simulink model "Vehicle_Model_999_Modular_roll_gradient"  (R2025b)
settings: Solver=ode23tb  StartTime=0.0  StopTime=72  MaxStep=0.001  RelTol=1e-3
values from neighbouring files (symbols this model uses):
  aero_par = struct()    [Load_aero_parameters.m]
  Ki_array = zeros(size(Vx_array))    [Torque_vectoring_workspace_lookuptable_v2.m]
  Kp_array = zeros(size(Vx_array))    [Torque_vectoring_workspace_lookuptable_v2.m]
  ku = (lr*m*9.81/(cf*(lf+lr))) - (lf*m*9.81/(cr*(lf+lr)))    (= -0.00172747958109)    [Torque_vectoring_workspace_lookuptable_v2.m]
  m = Par.m    [Lapsim_Endurance_inverse_v3.m]    (also in New_LapSim_final_ts_v1.m = Par.Mass; Rajdeep_sus_scriptv2.m = 270; Torque_vectoring_workspace_lookuptable_v2.m = 270)
  Par = struct()    [Load_vehicle_parameters.m]
  path_Theta = theta-theta_0    [New_LapSim_final_ts_v1.m]
  sus_par = struct()    [Load_sus_parameters.m]
  TireData = Tir    [prep_tire_data.m]
  Vx_array = 1:1:21    [Torque_vectoring_workspace_lookuptable_v2.m]
undefined symbols (not defined in the file or in its folder): additional_steering, Battery, Brake_Val, ctrl_Brake, ctrl_s, ctrl_Steer, ctrl_Throttle, ctrl_Velocity, HP, init_r, init_vx, init_vy, Motor, path_X, path_Y, skidpad_time, skidpad_vel, steer_input, Steer_Val, TC_target_slip, Throttle_Val, V_ref
libraries: simulink x16, autolibshared x3, simulink_extras x2, BatteryEstimators x1
(part 4 of 4)

== matlab function Vehicle_Model_999_Modular_roll_gradient/Vehicle dynamics/Fx, Fy calculations with grip limit/Grip_limit/MATLAB Function1 ==
  data: Fx input; Fx_new output; Fy input; Dx input; Dy input; s input; Fy_new output
function [Fx_new, Fy_new] = fcn(Fx, Fy, Dx, Dy, s)
    % Initialize outputs
    Fx_new = Fx;
    Fy_new = Fy;
    
    if s > 1
        % 1. Add a tiny protection value (1e-6) to prevent divide-by-zero
        Dx_safe = max(abs(Dx), 1e-3);
        Dy_safe = max(abs(Dy), 1e-3);
        
        % 2. Calculate the grip saturation (eta) for all tires
        eta = sqrt((Fx ./ Dx_safe).^2 + (Fy ./ Dy_safe).^2);
        
        % 3. Find the indices of the tires that are exceeding 100% grip
        over_limit_idx = eta > 1;
        
        % 4. Proportionally scale down ONLY the tires that are slipping
        % This scales the vector perfectly to the edge of the ellipse 
        % without changing the force direction.
        Fx_new(over_limit_idx) = Fx(over_limit_idx) ./ eta(over_limit_idx);
        Fy_new(over_limit_idx) = Fy(over_limit_idx) ./ eta(over_limit_idx);
    end
end

== matlab function Vehicle_Model_999_Modular_roll_gradient/E-powertrain/Motor/rpm selection for third wheel ==
  data: u input; y output
function y = fcn(u)

y = u(3);

== matlab function Vehicle_Model_999_Modular_roll_gradient/Inputs/steer_input_simulink/MATLAB Function ==
  settings: updateMethod=DISCRETE
  data: X input; delta output; Y input; PSI input; vx input; vy input; path_Y input; path_X input; path_Theta input
function delta = get_steering_command(X, Y, PSI, vx,vy,path_Y, path_X, path_Theta)
    % GET_STEERING_COMMAND Simulink-safe Stanley implementation
   
    %% Parameters
    L_f = 0.78132;          % Pre-multiplied 1.532 * 0.51 for efficiency
    v_eps = 1.0;            % Softening constant to prevent singularity
    v_switch = 5.0;         % Velocity threshold for slip compensation (m/s)
    max_steer = deg2rad(25);% Physical steering limit
    k_stanley = 0;
    %% 1. Sensing (Shift to Front Axle)
    xf = X + L_f * cos(PSI); 
    yf = Y + L_f * sin(PSI);
    
    %% 2. Global Nearest Point Search (Fixed-Size for Simulink)
    % Calculate squared distances to ALL points to maintain fixed array sizes
    dx = path_X - xf;
    dy = path_Y - yf;
    distances = dx.^2 + dy.^2; 
    
    [~, idx_closest] = min(distances);
    Npath = length(path_X);
    
    % %% 3. Path Heading Calculation
    % if Npath <= 1
    %     % Failsafe: If the path is only 1 point, we cannot calculate a slope.
    %     % Default to 0, or you could output an error flag.
    %     path_Theta = 0; 
    % elseif idx_closest < Npath
    %     % Forward difference (standard operation)
    %     path_Theta = atan2(path_X(idx_closest+1) - path_X(idx_closest),path_Y(idx_closest+1) - path_Y(idx_closest));
    % else
    %     % Backward difference (only triggers when exactly on the final point of the track)
    %     path_Theta = atan2(path_X(idx_closest) - path_X(idx_closest-1), path_Y(idx_closest) - path_Y(idx_closest-1));
    % end
    
    %% 4. Error Calculations
    % Crosstrack Error ($e_{ct}$)
    % Cross product mapping ensures right-hand rule sign convention is maintained
    e_ct = (path_Y(idx_closest) - yf)*cos(path_Theta) - (path_X(idx_closest) - xf)*sin(path_Theta);
    
    % Heading Error ($\theta_e$)
    % Wrapped strictly between [-pi, pi]
    theta_e = atan2(sin(path_Theta - PSI), cos(path_Theta - PSI));
    
    %Side_slip calculations:
    beta = atan2(vy,vx);
    
    %% 5. Control Law (Stanley)
    % $\delta = (\theta_e - \beta) + \arctan(k \cdot e_{ct} / (v_x + v_{eps}))$
    delta_raw = (theta_e - beta) + atan2(k_stanley * e_ct, vx + v_eps);
    
    % Apply physical steering limits
    delta = max(min(delta_raw, max_steer), -max_steer);
end

== matlab function Vehicle_Model_999_Modular_roll_gradient/Inputs/Subsystem1/MATLAB Function ==
  data: is_above input; count output
function count = count_crossings(is_above)
    % Initialize persistent variables to remember data between time steps
    persistent prev_state total_count
    
    % Initialize values on the very first time step
    if isempty(prev_state)
        prev_state = is_above; % Set to current state to avoid a false count at t=0
        total_count = 0;
    end
    
    % Detect if the state has changed (a crossing occurred)
    if is_above ~= prev_state
        total_count = total_count + 1;
        prev_state = is_above; % Update the stored state
    end
    
    % Output the current count
    count = total_count;
end

== matlab function Vehicle_Model_999_Modular_roll_gradient/Vehicle dynamics/Fx, Fy calculations with grip limit/MATLAB Function ==
  data: u input; y output
function y = fcn(u)

y = sum(u);

== matlab function Vehicle_Model_999_Modular_roll_gradient/Inputs/steer_input_simulink/Velocity iterations ==
  data: delta output; Par parameter; ku parameter; additional_steering input; skidpad_vel input
function delta = fcn(Par,ku,additional_steering, skidpad_vel)
R = 9.125;
distance = 2*pi*R;
vx = skidpad_vel;
skidpad_time = distance/skidpad_vel;
psi_dot = 2*pi/skidpad_time;   % yaw rate in rad/s for 5 sec skidpad

ku = ku/9.81;
delta = Par.WB*(psi_dot/vx) + ku*vx*psi_dot + additional_steering;

== matlab function Vehicle_Model_999_Modular_roll_gradient/E-powertrain/Torque Distribution/is TCS on?/MATLAB Function1 ==
  data: Steer_input input; TC_on output
function TC_on = fcn(Steer_input)
if abs(Steer_input) < rad2deg(7)
    TC_on = 1;
else 
    TC_on = 0;
end

== matlab function Vehicle_Model_999_Modular_roll_gradient/Vehicle dynamics/Steering/Steering Kinematics/Steering Kinematics ==
  data: Steer_Input input; Ackermann_Pct input; Steer_FL output; Steer_FR output; Par parameter
function [Steer_FL, Steer_FR] = fcn(Steer_Input, Ackermann_Pct, Par)
%#codegen

    % 1. Constants
    L = Par.WB;      % Wheelbase
    half_T = Par.TW / 2; % Half Track Width

    % 2. Safety Clamp (Prevent tan(90) singularity)
    delta = min(max(Steer_Input, -1.5), 1.5); 
    
    % 3. Calculate "Pure Ackermann" Angles
    % Ideally, inner wheel turns sharper than outer wheel.
    tan_d = tan(delta);
    
    % FL (Left): Denom depends on sign of turn.
    % If turning Left (+), Denom shrinks (Sharper).
    FL_Ack = atan( (L * tan_d) / (L - half_T * tan_d) );
    
    % FR (Right): 
    % If turning Left (+), Denom grows (Shallower).
    FR_Ack = atan( (L * tan_d) / (L + half_T * tan_d) );
    
    % 4. Calculate "Parallel" Angles
    % Both wheels exactly match the center input
    FL_Par = delta;
    FR_Par = delta;
    
    % 5. Linear Blend based on Percentage
    % Formula: Final = Parallel + (Ackermann - Parallel) * Percent
    Steer_FL = FL_Par + (FL_Ack - FL_Par) * Ackermann_Pct;
    Steer_FR = FR_Par + (FR_Ack - FR_Par) * Ackermann_Pct;

end

== matlab function Vehicle_Model_999_Modular_roll_gradient/Vehicle dynamics/Steering_new/Steering Kinematics ==
  data: steering_wheel_angle input; Steer_L output; Steer_R output
function [Steer_L, Steer_R] = calculate_wheel_angles(steering_wheel_angle)
    % --- Constants & User Geometry (Matched to CAD Sketch) ---
    d = 61.543;              % Rack offset (Y-distance from Kingpin axis)
    L = 351;                 % Tie rod length (Now strictly enforced per CAD)
    R = 61.3;                % Steering arm length (Updated from CAD)
    theta1 = 90 - 83.625;    % Steering arm neutral angle (6.375 deg from longitudinal)
    
    % Track Definitions derived from CAD
    track_width = 1235;      % True automotive track width (Wheel center to wheel center)
    spindle_length = 44.075; % Distance from kingpin to outer wheel center
    kingpin_track = track_width - 2 * spindle_length; % Calculate Kingpin track dynamically
    
    % --- Structural Reference Points ---
    % Kingpins (Fixed Pivot Points)
    lx_kp = -kingpin_track/2;
    rx_kp = kingpin_track/2;
    y_kp = d;
    y_rack = 0;
    
    % Neutral Rack Ends (Derived geometrically from Kingpins)
    lx_rack_neutral = lx_kp - R*sind(theta1) + sqrt(L^2 - (d - R*cosd(theta1))^2);
    rx_rack_neutral = rx_kp + R*sind(theta1) - sqrt(L^2 - (d - R*cosd(theta1))^2);
    
    % --- Steering Ratio Conversion ---
    % Convert Steering Wheel Angle (deg) to Rack Displacement (mm)
    % Update c_factor to match your actual pinion radius (mm travel per 1 deg of steering wheel)
    c_factor = 43.9267; 
    x_input = steering_wheel_angle * c_factor;
    
    % Initialize output arrays to support vector inputs
    num_inputs = length(x_input);
    Steer_L = zeros(num_inputs, 1);
    Steer_R = zeros(num_inputs, 1);
    
    % Calculate for each input angle
    for i = 1:num_inputs
        xi = x_input(i);
        
        % 1. Calculate strictly horizontal Rack ends
        lx_rack = lx_rack_neutral + xi;
        rx_rack = rx_rack_neutral + xi;
        
        % 2. Solve for Steering Arm Angles by enforcing exact Tie Rod Length (L)
        % Equation: (X_outer - X_rack)^2 + (Y_outer - Y_rack)^2 - L^2 = 0
        fun_L = @(t) (lx_kp - R*sind(t) - lx_rack)^2 + (y_kp - R*cosd(t) - y_rack)^2 - L^2;
        fun_R = @(t) (rx_kp + R*sind(t) - rx_rack)^2 + (y_kp - R*cosd(t) - y_rack)^2 - L^2;
        
        % Find the roots using the neutral angle as the initial guess
        tL = fzero(fun_L, theta1);
        tR = fzero(fun_R, theta1);
        
        % 3. Calculate absolute rotation of the knuckle assembly
        % Left wheel angle
        Steer_L(i) = deg2rad(theta1 - tL); 
        
        % Right wheel angle
        Steer_R(i) = deg2rad(tR - theta1); 
    end
end

== matlab function Vehicle_Model_999_Modular_roll_gradient/Vehicle dynamics/Suspension/MATLAB Function1 ==
  data: Lateral_accln input; Roll_angle output; sus_par parameter
function Roll_angle = fcn(Lateral_accln, sus_par)
g = 9.81;
Roll_angle = deg2rad(sus_par.Roll_gradient*Lateral_accln/g);
end

== matlab function Vehicle_Model_999_Modular_roll_gradient/Vehicle dynamics/Wheel_dynamics/Rolling Resistance ==
  data: Fz input; wFx_rr output; Omega input; slip_angles input; Par parameter
function wFx_rr  = fcn(Fz, Omega,slip_angles, Par)
%#codegen

    % 1. Calculate Total Magnitude
    F_mag = Par.C_rr .* abs(Fz);

    % 2. Determine Direction
    Dir = tanh(10 * Omega);

    
    % X-Component: Resists Spin (Torque generating)
    % wFx = -Magnitude * Direction * cos(Alpha)
    wFx_rr = -F_mag .*Dir.* cos(slip_angles);

end
